simulink model "DifferenceEquation_model"  (R2021a)
settings: Solver=FixedStepDiscrete  StartTime=0.0  StopTime=tFinal_s  FixedStep=T  RelTol=1e-3
settings Model: Creator=chris  LastModifiedBy=chris

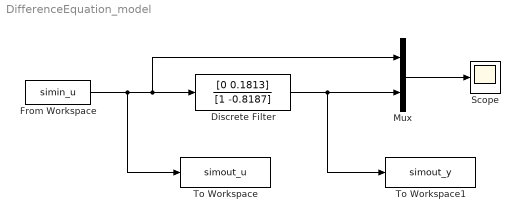
== system DifferenceEquation_model ==
  Discrete Filter : DiscreteFilter  Numerator=[0 0.1813]  Denominator=[1 -0.8187]
  From Workspace : FromWorkspace  VariableName=simin_u
  Mux : Mux  Inputs=2
  Scope : Scope
  To Workspace : ToWorkspace  VariableName=simout_u  SaveFormat=Timeseries  SampleTime=-1
  To Workspace1 : ToWorkspace  VariableName=simout_y  SaveFormat=Timeseries  SampleTime=-1
  wires:
  From Workspace/1 -> To Workspace/1, Mux/1, Discrete Filter/1
  Discrete Filter/1 -> To Workspace1/1, Mux/2
  Mux/1 -> Scope/1
